simulink model "contM"  (R2018b)
settings: Solver=FixedStepAuto  StartTime=0.0  StopTime=1.0  FixedStep=0.2  RelTol=1e-3  EnableMultiTasking=on
settings Model: Creator=Reichl  LastModifiedBy=Reichl
settings DataIOCC: FinalStateName=xFinalCont  SaveFinalState=on  SaveCompleteFinalSimState=on  SaveFormat=Array  SaveState=on  SaveTime=off  StateSaveName=xContStates
settings OptimizationCC: LifeSpan=inf
settings DebuggingCC: AllowSymbolicDim=off  SFUnexpectedBacktrackingDiag=warning  SFNoUnconditionalDefaultTransitionDiag=warning  SFExecutionAtInitializationDiag=none
settings ModelReferenceCC: PropagateSignalLabelsOutOfModel=off
settings SFSimCC: SimUseLocalCustomCode=off
settings RTWCC: RTWUseLocalCustomCode=off
settings CodeAppCC: StateflowObjectComments=on
settings GRTTargetCC: TargetLangStandard=C89/C90 (ANSI)
settings ConfigComp: CovMetricSettings=dw  CovHtmlReporting=on  CovSaveCumulativeToWorkspaceVar=on  CovSaveSingleToWorkspaceVar=on  CovExternalEMLEnable=off

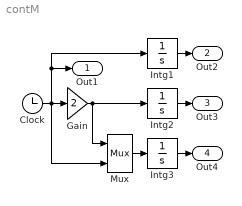
== system contM ==
  Clock : Clock
  Gain : Gain  Gain=2
  Intg1 : Integrator  ContinuousStateAttributes='x1'
  Intg2 : Integrator  ContinuousStateAttributes='x2'
  Intg3 : Integrator  ContinuousStateAttributes={ 'xa', 'xb' }
  Mux : Mux  Inputs=2
  Out1 : Outport
  Out2 : Outport  Port=2
  Out3 : Outport  Port=3
  Out4 : Outport  Port=4
  wires:
  Clock/1 -> Intg1/1, Out1/1, Gain/1, Mux/2
  Intg1/1 -> Out2/1
  Intg2/1 -> Out3/1
  Intg3/1 -> Out4/1
  Gain/1 -> Intg2/1, Mux/1
  Mux/1 -> Intg3/1
